simulink model "pneumatic_tank_sysid"  (R2018b)
settings: Solver=ode15s  StartTime=0.0  StopTime=60  FixedStep=1e-3  RelTol=1e-3
PreLoadFcn:
  | delta_p = 0.6; % MPa
  | p_init = 0.101325; % MPa
  | T_init = 293.15; % K
  | T_atm = 293.15; % K
  | 
  | A_valve_max = 4e-6; % m^2
  | A_valve_min = 1e-10; % m^2
  | 
  | A_pipe = 5e-6; % m^2
  | L_pipe = 1; % m
  | 
  | A_piston = 0.002; % m^2
  | L_piston = 0.2; % m
libraries: fl_lib x31, nesl_utility x6
(part 1 of 3)
CloseFcn:
  | try,close(h1_ssc_pneumatic_actuator),end
  | clear h1_ssc_pneumatic_actuator
  | try,close(h2_ssc_pneumatic_actuator),end
  | clear h2_ssc_pneumatic_actuator
  | 
  | clear simlog_ssc_pneumatic_actuator tout
  | clear delta_p p_init T_init T_atm
  | clear A_valve_max A_valve_min
  | clear A_pipe L_pipe A_piston L_piston load
Description:
  | Pneumatic Actuation Circuit
  | 
  | Copyright 2016-2018 The MathWorks, Inc.
settings Model: Creator=MathWorks  LastModifiedBy=kjartan
settings DebuggingCC: LibraryContextMissingDiagnostic=none
settings SFSimCC: SimUseLocalCustomCode=off
settings RTWCC: RTWUseLocalCustomCode=off
settings CodeAppCC: StateflowObjectComments=on
settings GRTTargetCC: TargetLangStandard=C89/C90 (ANSI)
settings ConfigComp: CovMetricSettings=dsw  CovHtmlReporting=on  CovSaveCumulativeToWorkspaceVar=on  CovSaveSingleToWorkspaceVar=on  CovShowResultsExplorer=off  CovExternalEMLEnable=off
settings SimscapeCC: SimscapeNominalValues="[{\"value\":\"1\",\"unit\":\"A\"},{\"value\":\"1\",\"unit\":\"bar\"},{\"value\":\"1\",\"unit\":\"cm^2\"},{\"value\":\"1\",\"unit\":\"cm^3/s\"},{\"value\":\"500\",\"unit\":\"kJ/kg\"},{\"value\":\"1\",\"unit\":\"kW\"},{\"value\":\"1\",\"unit\":\"l\"},{\"value\":\"1\",\"unit\":\"N\"},{\"value\":\"1\",\"unit\":\"N*m\"},{\"value\":\"1\",\"unit\":\"V\"}]"  SimscapeLogType=all  SimscapeLogSimulationStatistics=on  SimscapeLogName=simlog_ssc_pneumatic_actuator  SimscapeLogDataHistory=10000

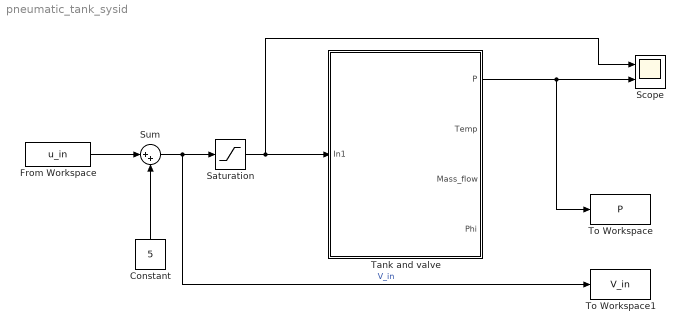
== system pneumatic_tank_sysid ==
  Constant : Constant  Value=5
  From Workspace : FromWorkspace  VariableName=u_in  SampleTime=0  OutputAfterFinalValue=Holding final value
  Saturation : Saturate  UpperLimit=10  LowerLimit=0
  Scope : Scope  NumInputPorts=2
  Sum : Sum  Inputs=|++
  Tank and valve : Subsystem
  To Workspace : ToWorkspace  VariableName=P  SaveFormat=Timeseries  SampleTime=-1
  To Workspace1 : ToWorkspace  VariableName=V_in  SaveFormat=Timeseries  SampleTime=-1
  wires:
  Tank and valve/1(P) -> To Workspace/1, Scope/2
  Constant/1 -> Sum/2
  Sum/1 -> To Workspace1/1, Saturation/1  "V_in"
  From Workspace/1 -> Sum/1
  Saturation/1 -> Scope/1, Tank and valve/1(In1)
